simulink model "CaptureOutputs"  (R2018b)
settings: Solver=ode4  StartTime=0.0  StopTime=SimEndTime  FixedStep=TimeStep  RelTol=1e-3
model workspace (MATLAB code in the model file):
  | CON = Simulink.Parameter;
  | CON.DataType = 'Bus: Bus_CON';
  | CON.Value = Simulink.Bus.createMATLABStruct('Bus_CON');
undefined symbols (not defined in the file): SampleTime
settings Model: ParameterArgumentNames=CON  OrderedModelArguments=off  Creator=Ethan  LastModifiedBy=Ethan
settings ModelReferenceCC: ModelReferenceNumInstancesAllowed=Single

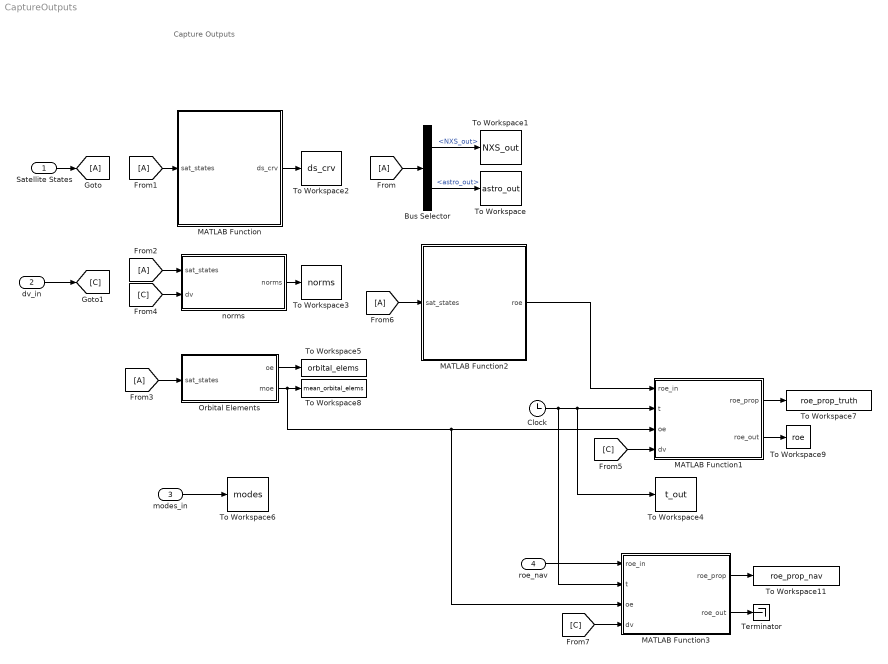
== system CaptureOutputs ==
  note: Capture Outputs
  Satellite States : Inport  OutDataTypeStr=Bus: Bus_outputs
  dv_in : Inport  Port=2  PortDimensions=3
  modes_in : Inport  Port=3  OutDataTypeStr=Bus: Bus_modes
  roe_nav : Inport  Port=4  OutDataTypeStr=Bus: Bus_roe
  Bus Selector : BusSelector  OutputSignals=NXS_out,astro_out
  Clock : Clock
  MATLAB Function : MATLAB Function  TreatAsAtomicUnit=on
  MATLAB Function1 : MATLAB Function  TreatAsAtomicUnit=on  SystemSampleTime=SampleTime
  MATLAB Function2 : MATLAB Function  TreatAsAtomicUnit=on
  MATLAB Function3 : MATLAB Function  TreatAsAtomicUnit=on  SystemSampleTime=SampleTime
  Orbital Elements : MATLAB Function  TreatAsAtomicUnit=on
  Terminator : Terminator
  To Workspace : ToWorkspace  VariableName=astro_out  SampleTime=SampleTime
      settings: Save2DSignal=2-D array (concatenate along first dimension)
  To Workspace1 : ToWorkspace  VariableName=NXS_out  SampleTime=SampleTime
      settings: Save2DSignal=2-D array (concatenate along first dimension)
  To Workspace11 : ToWorkspace  VariableName=roe_prop_nav  SaveFormat=Timeseries  SampleTime=SampleTime
      settings: Save2DSignal=2-D array (concatenate along first dimension)
  To Workspace2 : ToWorkspace  VariableName=ds_crv  SampleTime=SampleTime
      settings: Save2DSignal=2-D array (concatenate along first dimension)
  To Workspace3 : ToWorkspace  VariableName=norms  SaveFormat=Timeseries  SampleTime=SampleTime
      settings: Save2DSignal=2-D array (concatenate along first dimension)
  To Workspace4 : ToWorkspace  VariableName=t_out  SampleTime=SampleTime
      settings: Save2DSignal=2-D array (concatenate along first dimension)
  To Workspace5 : ToWorkspace  VariableName=orbital_elems  SaveFormat=Timeseries  SampleTime=SampleTime
      settings: Save2DSignal=2-D array (concatenate along first dimension)
  To Workspace6 : ToWorkspace  VariableName=modes  SaveFormat=Timeseries  SampleTime=SampleTime
      settings: Save2DSignal=2-D array (concatenate along first dimension)
  To Workspace7 : ToWorkspace  VariableName=roe_prop_truth  SaveFormat=Timeseries  SampleTime=SampleTime
      settings: Save2DSignal=2-D array (concatenate along first dimension)
  To Workspace8 : ToWorkspace  VariableName=mean_orbital_elems  SaveFormat=Timeseries  SampleTime=SampleTime
      settings: Save2DSignal=2-D array (concatenate along first dimension)
  To Workspace9 : ToWorkspace  VariableName=roe  SaveFormat=Timeseries  SampleTime=SampleTime
      settings: Save2DSignal=2-D array (concatenate along first dimension)
  norms : MATLAB Function  TreatAsAtomicUnit=on
  wires:
  Satellite States/1 -> [A]
  MATLAB Function/1(ds_crv) -> To Workspace2/1
  [A] -> Bus Selector/1
  Bus Selector/2 -> To Workspace/1  "<astro_out>"
  Bus Selector/1 -> To Workspace1/1  "<NXS_out>"
  norms/1(norms) -> To Workspace3/1
  [A] -> MATLAB Function/1(sat_states)
  [A] -> norms/1(sat_states)
  [A] -> Orbital Elements/1(sat_states)
  Orbital Elements/1(oe) -> To Workspace5/1
  modes_in/1 -> To Workspace6/1
  MATLAB Function2/1(roe) -> MATLAB Function1/1(roe_in)
  Orbital Elements/2(moe) -> MATLAB Function3/3(oe), MATLAB Function1/3(oe), To Workspace8/1
  MATLAB Function1/1(roe_prop) -> To Workspace7/1
  MATLAB Function1/2(roe_out) -> To Workspace9/1
  dv_in/1 -> [C]
  [C] -> norms/2(dv)
  [C] -> MATLAB Function1/4(dv)
  [A] -> MATLAB Function2/1(sat_states)
  MATLAB Function3/1(roe_prop) -> To Workspace11/1
  Clock/1 -> MATLAB Function3/2(t), To Workspace4/1, MATLAB Function1/2(t)
  [C] -> MATLAB Function3/4(dv)
  MATLAB Function3/2(roe_out) -> Terminator/1
  roe_nav/1 -> MATLAB Function3/1(roe_in)

== matlab function CaptureOutputs/norms ==
  data: sat_states input; norms output Bus: Bus_sat_norms; dv input
function norms = norm_outputs(sat_states, dv)

NXS = sat_states.NXS_out;
astro = sat_states.astro_out;


norms.NXS.r = norm(NXS.r_i);
norms.astro.r = norm(astro.r_i);
norms.NXS.v = norm(NXS.v_i);
norms.astro.v = norm(astro.v_i);
norms.dv = norm(dv);
end

== matlab function CaptureOutputs/MATLAB Function ==
  data: sat_states input; ds_crv output
function ds_crv  = i2relRTN(sat_states)
    rTgt = sat_states.NXS_out.r_i;
    vTgt = sat_states.NXS_out.v_i;
    rChase = sat_states.astro_out.r_i;
    vChase = sat_states.astro_out.v_i;
    [rHill,vHill] = ECI2Hill_Vectorized(rTgt,vTgt,rChase,vChase);
    ds_crv = [rHill; vHill];
end

== matlab function CaptureOutputs/Orbital Elements ==
  data: sat_states input; oe output Bus: Bus_sat_oe; CON parameter; moe output Bus: Bus_sat_oe
function [oe, moe] = orbital_elements(sat_states, CON)


NXS = sat_states.NXS_out;
astro = sat_states.astro_out;

[oe.NXS.a, oe.NXS.e, oe.NXS.inc, oe.NXS.omega, oe.NXS.w, oe.NXS.nu]...
    = ECI2OE(NXS.r_i, NXS.v_i, CON.mu);
[oe.astro.a, oe.astro.e, oe.astro.inc, oe.astro.omega, oe.astro.w, oe.astro.nu]... 
    = ECI2OE(astro.r_i, astro.v_i, CON.mu);

moe_NXS = osc2mean([oe.NXS.a, oe.NXS.e, oe.NXS.inc, oe.NXS.omega, oe.NXS.w, oe.NXS.nu], CON.Re, CON.J2);

moe.NXS.a = moe_NXS(1);
moe.NXS.e = moe_NXS(2);
moe.NXS.inc = moe_NXS(3);
moe.NXS.omega = moe_NXS(4);
moe.NXS.w = moe_NXS(5);
moe.NXS.nu = moe_NXS(6);

moe_astro = osc2mean([oe.astro.a, oe.astro.e, oe.astro.inc, oe.astro.omega, oe.astro.w, oe.astro.nu], CON.Re, CON.J2);

moe.astro.a = moe_astro(1);
moe.astro.e = moe_astro(2);
moe.astro.inc = moe_astro(3);
moe.astro.omega = moe_astro(4);
moe.astro.w = moe_astro(5);
moe.astro.nu = moe_astro(6);
end

== matlab function CaptureOutputs/MATLAB Function1 ==
  settings: updateMethod=DISCRETE
  data: roe_in input; roe_prop output; t input; oe input; dv input; CON parameter; roe_out output Bus: Bus_roe
function [roe_prop, roe_out] = roe_prop(roe_in, t, oe, dv, CON)

reset_flag = 0;
persistent t0 roe_0
if isempty(t0)
    t0 = t;
    roe_0 = [roe_in.adot, roe_in.da, roe_in.dL, roe_in.dex, roe_in.dey, roe_in.dix, roe_in.diy];
end
if t == CON.SampleTime
    t0 = t;
    roe_0 = [roe_in.adot, roe_in.da, roe_in.dL, roe_in.dex, roe_in.dey, roe_in.dix, roe_in.diy];
end

if any(dv ~= zeros(3, 1))
    t0 = t;
    roe_0 = [roe_in.adot, roe_in.da, roe_in.dL, roe_in.dex, roe_in.dey, roe_in.dix, roe_in.diy];
    reset_flag = 1;
end

eta = sqrt(1 - oe.NXS.e^2);
gamma = CON.J2/2 * (CON.Re / oe.NXS.a)^2 * (1 / eta^4);
nc = sqrt(CON.mu / oe.NXS.a^3);

A = roe_state_matrix(nc, t - t0, oe.NXS, gamma, reset_flag, CON);

roe_prop = A * roe_0';
roe_out = roe_in;

== matlab function CaptureOutputs/MATLAB Function2 ==
  data: sat_states input; roe output Bus: Bus_roe; CON parameter
function roe  = i2roe(sat_states, CON)
persistent da_prev

chief = sat_states.NXS_out;
deputy = sat_states.astro_out;
% [ac,ec,ic,oc,wc,~, uc] = rvECI2oe_rad(chief.r_i, chief.v_i, CON.mu);
% [ad,ed,id,od,wd,~, ud] = rvECI2oe_rad(deputy.r_i, deputy.v_i, CON.mu);

[ac, ec, ic, oc, wc, ~, uc] = ECI2OE(chief.r_i, chief.v_i, CON.mu);
[ad, ed, id, od, wd, ~, ud] = ECI2OE(deputy.r_i, deputy.v_i, CON.mu);
deg2rad = pi / 180;
ic = ic * deg2rad;
oc = oc * deg2rad;
wc = wc * deg2rad;
uc = uc * deg2rad;

id = id * deg2rad;
od = od * deg2rad;
wd = wd * deg2rad;
ud = ud * deg2rad;

if sign(chief.r_i(3)) ~= sign(deputy.r_i(3))
    if sign(chief.r_i(3)) == -1
%         uc = uc - 2 * pi;
    else
        ud = ud - 2 * pi;
    end
end
if isempty(da_prev)
    da_prev = (ad - ac) / ac;
end

% moe_c = osc2mean([ac,ec,ic,oc,wc, uc], CON.Re, CON.J2);
% moe_d = osc2mean([ad,ed,id,od,wd, ud] , CON.Re, CON.J2);


roe.adot = -4.5075e-10;
roe.da = (ad - ac) / ac;
roe.dL = (ud - uc) + (od - oc) * cos(ic);
roe.dex = ed * cos(wd) - ec * cos(wc);
roe.dey = ed * sin(wd) - ec * sin(wc);
roe.dix = id - ic;
roe.diy = (od - oc) * sin(ic);

% roetemp = oe2roe(moe_c, moe_d, 1);
% 
% roe.adot = (roetemp(1) - da_prev) / CON.computer_dt;
% roe.da = roetemp(1);
% roe.dL = roetemp(2);
% roe.dex = roetemp(3);
% roe.dey = roetemp(4);
% roe.dix = roetemp(5);
% roe.diy = roetemp(6);
da_prev = roe.da;
end

== matlab function CaptureOutputs/MATLAB Function3 ==
  settings: updateMethod=DISCRETE
  data: roe_in input; roe_prop output; t input; oe input; dv input; CON parameter; roe_out output Bus: Bus_roe
function [roe_prop, roe_out] = roe_prop(roe_in, t, oe, dv, CON)

reset_flag = 0;
persistent t0 roe_0
if isempty(t0)
    t0 = t;
    roe_0 = [roe_in.adot, roe_in.da, roe_in.dL, roe_in.dex, roe_in.dey, roe_in.dix, roe_in.diy];
end
if t == 1 * CON.SampleTime
    t0 = t;
    roe_0 = [roe_in.adot, roe_in.da, roe_in.dL, roe_in.dex, roe_in.dey, roe_in.dix, roe_in.diy];
end

if any(dv ~= zeros(3, 1))
    t0 = t;
    roe_0 = [roe_in.adot, roe_in.da, roe_in.dL, roe_in.dex, roe_in.dey, roe_in.dix, roe_in.diy];
    reset_flag = 1;
end

eta = sqrt(1 - oe.NXS.e^2);
gamma = CON.J2/2 * (CON.Re / oe.NXS.a)^2 * (1 / eta^4);
nc = sqrt(CON.mu / oe.NXS.a^3);

A = roe_state_matrix(nc, t - t0, oe.NXS, gamma, reset_flag, CON);

roe_prop = A * roe_0';
roe_out = roe_in;
